simulink model "Subsystem_saturation"  (R2020a)
settings: Solver=VariableStepAuto  StartTime=0.0  StopTime=100.0  RelTol=1e-3
libraries: simulink x1
settings Model: Creator=109813  LastModifiedBy=109813

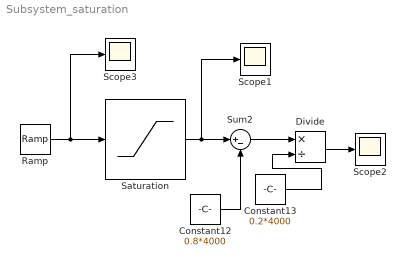
== system Subsystem_saturation ==
  Constant12 : Constant  Value=0.8*4000
  Constant13 : Constant  Value=0.2*4000
  Divide : Product  Inputs=*/
  Ramp : simulink/Sources/Ramp  slope=100  start=0  InitialOutput=0
  Saturation : Saturate  UpperLimit=4000  LowerLimit=4000*0.8
  Scope1 : Scope
  Scope2 : Scope
  Scope3 : Scope
  Sum2 : Sum  Inputs=|+-
  wires:
  Saturation/1 -> Scope1/1, Sum2/1
  Constant12/1 -> Sum2/2
  Constant13/1 -> Divide/2
  Divide/1 -> Scope2/1
  Ramp/1 -> Scope3/1, Saturation/1
  Sum2/1 -> Divide/1
